simulink model "Project3a"  (R2016a)
settings: Solver=ode5  StartTime=0.0  StopTime=tf  FixedStep=0.001  RelTol=1e-3
values from neighbouring files (symbols this model uses):
  k1 = 1    [Project3_FullCode.m]    (also in Project3a_Code.m = 30; Project3b_Code.m)
  k2 = 1    [Project3_FullCode.m]    (also in Project3a_Code.m = 40; Project3b_Code.m)
  k3 = 10    [Project3_FullCode.m]    (also in Project3a_Code.m)
  ugain = 1    [Project3_FullCode.m]    (also in Project3a_Code.m; Project3b_Code.m)
  x10 = 0    [Project3_FullCode.m]    (also in Project3a_Code.m = 1; Project3b_Code.m)
  x20 = 2    [Project3_FullCode.m]    (also in Project3a_Code.m = 0; Project3b_Code.m)
  x30 = 0    [Project3_FullCode.m]    (also in Project3a_Code.m)
settings Model: Creator=Dell  LastModifiedBy=Dell

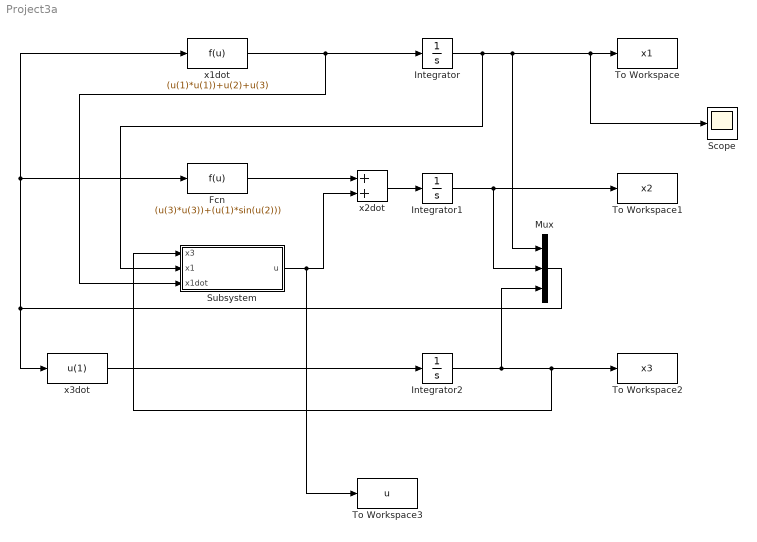
== system Project3a ==
  Fcn : Fcn  Expr=(u(3)*u(3))+(u(1)*sin(u(2)))
  Integrator : Integrator  InitialCondition=x10
  Integrator1 : Integrator  InitialCondition=x20
  Integrator2 : Integrator  InitialCondition=x30
  Mux : Mux  Inputs=3
  Scope : Scope
  Subsystem : Subsystem
  To Workspace : ToWorkspace  VariableName=x1  SampleTime=-1
  To Workspace1 : ToWorkspace  VariableName=x2  SampleTime=-1
  To Workspace2 : ToWorkspace  VariableName=x3  SampleTime=-1
  To Workspace3 : ToWorkspace  VariableName=u  SampleTime=-1
  x1dot : Fcn  Expr=(u(1)*u(1))+u(2)+u(3)
  x2dot : Sum
  x3dot : Fcn  Expr=u(1)
  wires:
  Integrator/1 -> Subsystem/2(x1), Mux/1, Scope/1, To Workspace/1
  Integrator1/1 -> Mux/2, To Workspace1/1
  Integrator2/1 -> Mux/3, Subsystem/1(x3), To Workspace2/1
  x1dot/1 -> Subsystem/3(x1dot), Integrator/1
  Mux/1 -> x3dot/1, Fcn/1, x1dot/1
  x3dot/1 -> Integrator2/1
  x2dot/1 -> Integrator1/1
  Subsystem/1(u) -> To Workspace3/1, x2dot/2
  Fcn/1 -> x2dot/1

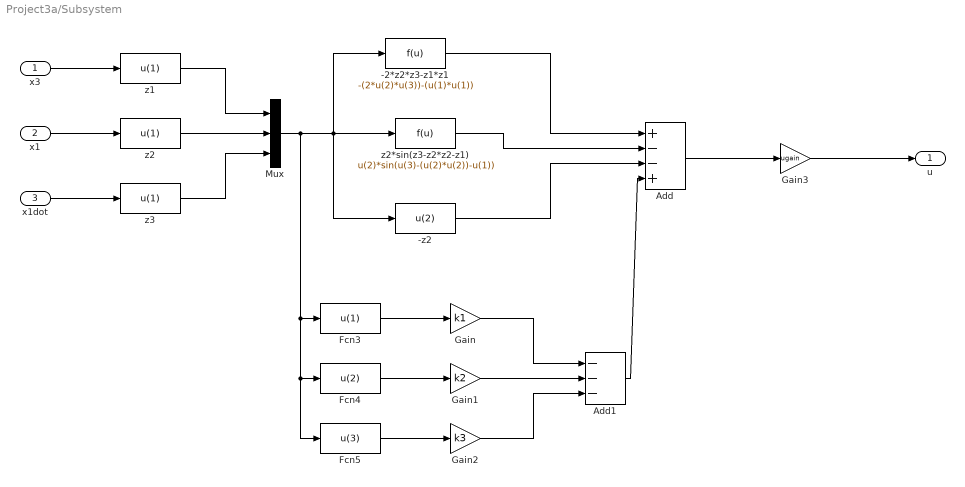
== system Project3a/Subsystem ==
  x3 : Inport
  x1 : Inport  Port=2
  x1dot : Inport  Port=3
  -2*z2*z3-z1*z1 : Fcn  Expr=-(2*u(2)*u(3))-(u(1)*u(1))
  -z2 : Fcn  Expr=u(2)
  Add : Sum  Inputs=+--+
  Add1 : Sum  Inputs=---
  Fcn3 : Fcn  Expr=u(1)
  Fcn4 : Fcn  Expr=u(2)
  Fcn5 : Fcn  Expr=u(3)
  Gain : Gain  Gain=k1
  Gain1 : Gain  Gain=k2
  Gain2 : Gain  Gain=k3
  Gain3 : Gain  Gain=ugain
  Mux : Mux  Inputs=3
  z1 : Fcn  Expr=u(1)
  z2 : Fcn  Expr=u(1)
  z2*sin(z3-z2*z2-z1) : Fcn  Expr=u(2)*sin(u(3)-(u(2)*u(2))-u(1))
  z3 : Fcn  Expr=u(1)
  u : Outport
  wires:
  x3/1 -> z1/1
  x1/1 -> z2/1
  x1dot/1 -> z3/1
  z1/1 -> Mux/1
  z2/1 -> Mux/2
  z3/1 -> Mux/3
  Mux/1 -> Fcn5/1, Fcn4/1, Fcn3/1, -z2/1, -2*z2*z3-z1*z1/1, z2*sin(z3-z2*z2-z1)/1
  -2*z2*z3-z1*z1/1 -> Add/1
  z2*sin(z3-z2*z2-z1)/1 -> Add/2
  -z2/1 -> Add/3
  Fcn3/1 -> Gain/1
  Fcn4/1 -> Gain1/1
  Fcn5/1 -> Gain2/1
  Gain1/1 -> Add1/2
  Gain/1 -> Add1/1
  Gain2/1 -> Add1/3
  Add1/1 -> Add/4
  Add/1 -> Gain3/1
  Gain3/1 -> u/1
